simulink model "Flight_Model_2015a_07_13_2020"  (R2015a)
settings: Solver=ode45  StartTime=0.0  StopTime=120  RelTol=1e-3
model workspace (MAT data in the model file):
  rocketDiam = 0.197
  noseLength = 0.5
  totalImpulse = 10831
  finSpan = 0.4
  finArea = 0.2
  finChordAngle = 0.5236
  refArea = 0.0182
  rocketCP = 1
  bodyLength = 5
  propMass = 7.183
  gravity = 9.8067
  time = [0; 0.045; 0.067; 0.084; 0.124; 0.186; 0.231; 0.298; 0.371; 0.534; 0.979; 1.142; 2.002; 2.289; 2.761; 3.121; 3.436; 3.678; 3.79; 4.004; 4.415; 4.538; 4.656; 4.82; 5.005; 5.219; 5.371]
  thrust = [0; 2638.366; 2528.97; 3063.078; 2426.009; 2548.275; 2599.755; 2554.71; 2644.801; 2638.366; 2561.145; 2606.19; 2638.366; 2638.366; 2580.45; 2496.795; 2335.919; 2213.653; 2129.998; 1653.805; 888.035; 630.634; 450.453; 289.577; 135.136; 25.74; 0]
  wetCG = 2.1
  dryCG = 1.9
  wetMass = 30
  dryMass = 23
  brakesOn = 1
  vehicleCd = 0.8
  fullBrakesOn = 0
  brakesCd = 1
  targetAlt = 3048
undefined symbols (not defined in the file): Earth, WGS84
libraries: aerolibasang x4, aerolibbdyn x3, aerolibwind2 x2, aerolib6dof2 x2, aerospace x1, aerolibtransform2 x1, aerolibfltsims x1, aerolibatmos2 x1
settings Model: Creator=jacob  LastModifiedBy=alhus

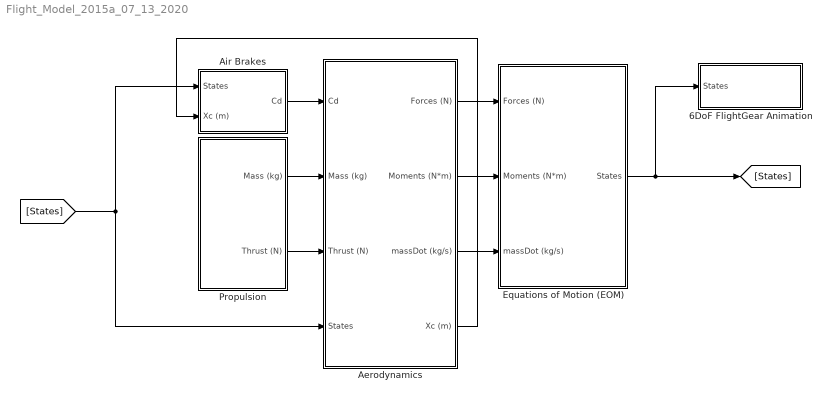
== system Flight_Model_2015a_07_13_2020 ==
  6DoF FlightGear Animation : Subsystem
  Aerodynamics : Subsystem
  Air Brakes : Subsystem
  Equations of Motion (EOM) : Subsystem
  Propulsion : Subsystem
  wires:
  Aerodynamics/1(Forces (N)) -> Equations of Motion (EOM)/1(Forces (N))
  Aerodynamics/2(Moments (N*m)) -> Equations of Motion (EOM)/2(Moments (N*m))
  Propulsion/1(Mass (kg)) -> Aerodynamics/2(Mass (kg))
  Propulsion/2(Thrust (N)) -> Aerodynamics/3(Thrust (N))
  Air Brakes/1("Cd ") -> Aerodynamics/1(Cd)
  Equations of Motion (EOM)/1(States) -> [States], 6DoF FlightGear Animation/1(States)
  [States] -> Air Brakes/1(States), Aerodynamics/4(States)
  Aerodynamics/3(massDot (kg/s)) -> Equations of Motion (EOM)/3(massDot (kg/s))
  Aerodynamics/4(Xc (m)) -> Air Brakes/2(Xc (m))

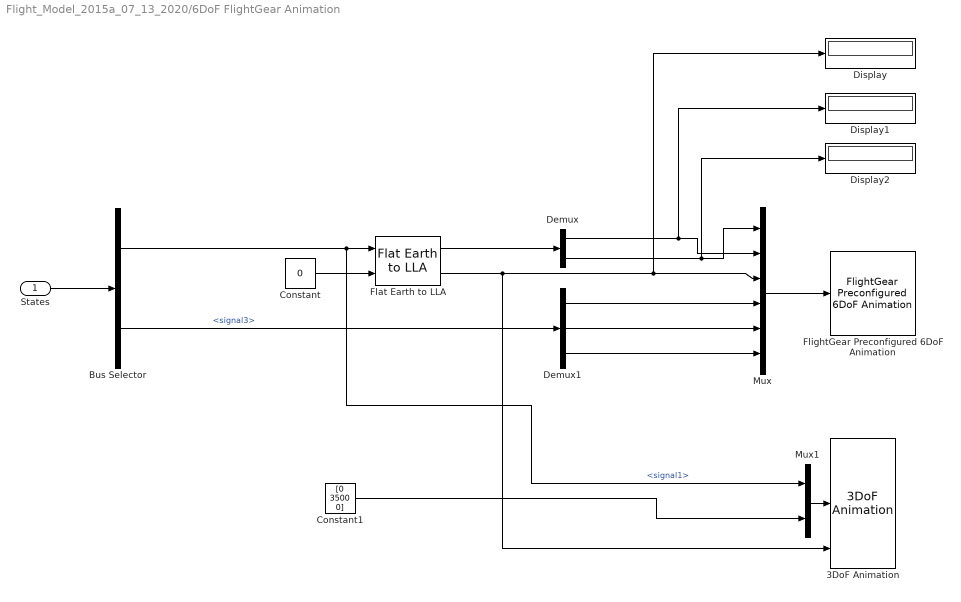
== system Flight_Model_2015a_07_13_2020/6DoF FlightGear Animation ==
  States : Inport
  3DoF Animation : aerospace/Animation/3DoF Animation  u1=[0 5000 -2000 2000 -5050 -3050]  u2=0.03  u3=1.8  u5=Fly alongside  u6=[200 200 -50]  u7=20  u8=on
  Bus Selector : BusSelector  OutputSignals=signal1,signal3
  Constant : Constant  Value=0
  Constant1 : Constant  Value=[0 3500 0]
  Demux : Demux  Outputs=2
  Demux1 : Demux  Outputs=3
  Display : Display
  Display1 : Display
  Display2 : Display
  Flat Earth to LLA : aerolibtransform2/Flat Earth to LLA  units=Metric (MKS)  ptype=Earth (WGS84)  F=1/298.257223563  R=6378137  LL0=[0 10]  psi=0
  FlightGear Preconfigured 6DoF Animation : aerolibfltsims/FlightGear Preconfigured 6DoF Animation  xFlightGearVersion=v3.0  DestinationIpAddress=127.0.0.1  DestinationPort=5502  SampleTime=1/30
  Mux : Mux  Inputs=6
  Mux1 : Mux  Inputs=2
  wires:
  States/1 -> Bus Selector/1
  Constant/1 -> Flat Earth to LLA/2
  Mux/1 -> FlightGear Preconfigured 6DoF Animation/1
  Flat Earth to LLA/1 -> Demux/1
  Demux/1 -> Display1/1, Mux/2
  Demux/2 -> Display2/1, Mux/1
  Flat Earth to LLA/2 -> 3DoF Animation/3, Display/1, Mux/3
  Demux1/2 -> Mux/5
  Demux1/3 -> Mux/6
  Demux1/1 -> Mux/4
  Bus Selector/1 -> Mux1/1, Flat Earth to LLA/1  "<signal1>"
  Bus Selector/2 -> Demux1/1  "<signal3>"
  Mux1/1 -> 3DoF Animation/2
  Constant1/1 -> Mux1/2

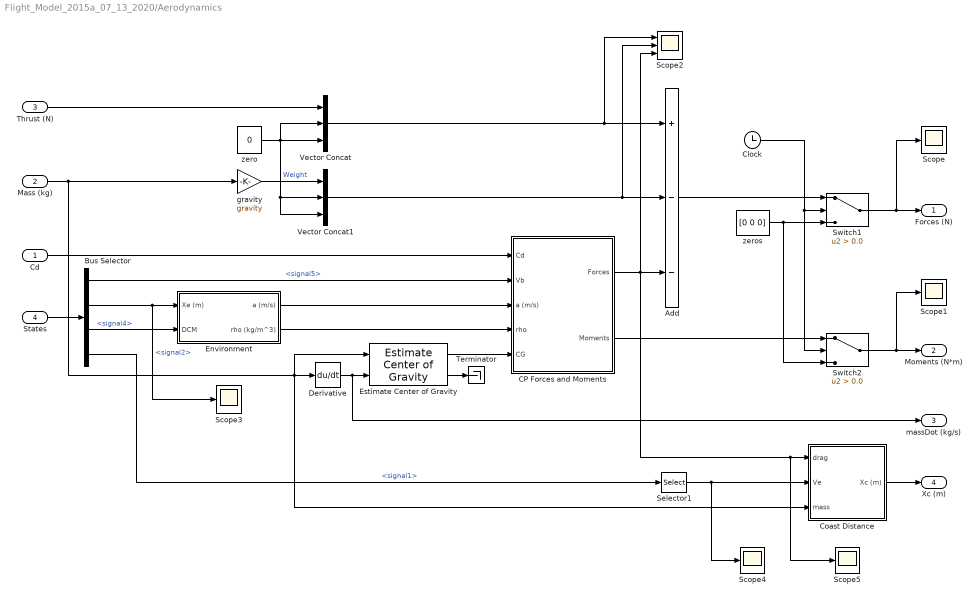
== system Flight_Model_2015a_07_13_2020/Aerodynamics ==
  Cd : Inport
  Mass (kg) : Inport  Port=2
  Thrust (N) : Inport  Port=3
  States : Inport  Port=4
  Add : Sum  Inputs=+--
  Bus Selector : BusSelector  OutputSignals=signal5,signal2,signal4,signal1
  CP Forces and Moments : Subsystem
  Clock : Clock
  Coast Distance : Subsystem
  Derivative : Derivative
  Environment : Subsystem
  Estimate Center of Gravity : aerolibbdyn/Estimate Center of Gravity  fmass=wetMass  emass=dryMass  fcg=[wetCG 0 0]'  ecg=[dryCG 0 0]'
  Scope{,1,3..5} (5 alike) : Scope
      Scope settings: YMin=-1  YMax=1  SaveName=ScopeData10
      Scope1 settings: SaveName=ScopeData11
      Scope3 settings: SaveName=ScopeData18
      Scope4 settings: SaveName=ScopeData20
      Scope5 settings: SaveName=ScopeData21
  Scope2 : Scope  NumInputPorts=3
      settings: YMin=-5~-5~-5  YMax=5~5~5  SaveName=ScopeData14
  Selector1 : Selector  InputPortWidth=3
  Switch1 : Switch  Criteria=u2 > Threshold  Threshold=0.0
  Switch2 : Switch  Criteria=u2 > Threshold  Threshold=0.0
  Terminator : Terminator
  Vector Concat : Concatenate  NumInputs=3
  Vector Concat1 : Concatenate  NumInputs=3
  gravity : Gain  Gain=gravity
  "zero " : Constant  Value=0
  "zeros " : Constant  Value=[0 0 0]
  Forces (N) : Outport
  Moments (N*m) : Outport  Port=2
  massDot (kg/s) : Outport  Port=3
  Xc (m) : Outport  Port=4
  wires:
  Mass (kg)/1 -> Coast Distance/3(mass), Estimate Center of Gravity/1, Derivative/1, gravity/1
  Derivative/1 -> Estimate Center of Gravity/2, massDot (kg/s)/1
  Estimate Center of Gravity/2 -> Terminator/1
  Estimate Center of Gravity/1 -> CP Forces and Moments/5(CG)
  Cd/1 -> CP Forces and Moments/1(Cd)
  Environment/2(rho (kg/m^3)) -> CP Forces and Moments/4(rho)
  Add/1 -> Switch1/1
  Switch1/1 -> Scope/1, Forces (N)/1
  "zeros "/1 -> Switch2/3, Switch1/3
  Clock/1 -> Switch2/2, Switch1/2
  Switch2/1 -> Scope1/1, Moments (N*m)/1
  States/1 -> Bus Selector/1
  Environment/1(a (m/s)) -> CP Forces and Moments/3(a (m/s))
  Bus Selector/1 -> CP Forces and Moments/2(Vb)  "<signal5>"
  Bus Selector/2 -> Environment/1(Xe (m)), Scope3/1  "<signal2>"
  Bus Selector/3 -> Environment/2(DCM)  "<signal4>"
  "zero "/1 -> Vector Concat/2, Vector Concat/3, Vector Concat1/2, Vector Concat1/3
  Thrust (N)/1 -> Vector Concat/1
  Vector Concat/1 -> Scope2/1, Add/1
  Vector Concat1/1 -> Scope2/2, Add/2
  CP Forces and Moments/2(Moments) -> Switch2/1
  gravity/1 -> Vector Concat1/1  "Weight"
  CP Forces and Moments/1(Forces) -> Scope5/1, Coast Distance/1(drag), Add/3, Scope2/3
  Bus Selector/4 -> Selector1/1  "<signal1>"
  Coast Distance/1(Xc (m)) -> Xc (m)/1
  Selector1/1 -> Coast Distance/2(Ve), Scope4/1

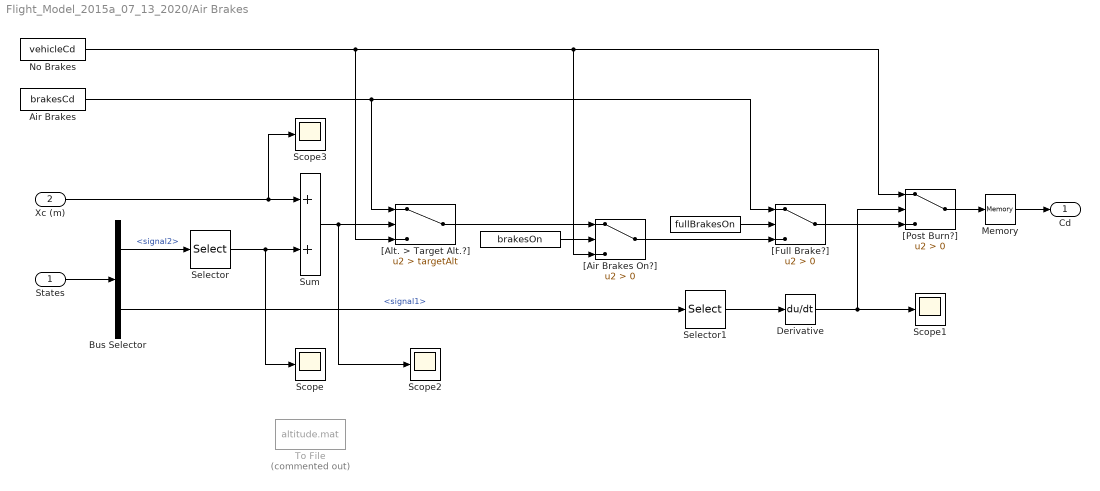
== system Flight_Model_2015a_07_13_2020/Air Brakes ==
  States : Inport
  Xc (m) : Inport  Port=2
  " " : Constant  Value=fullBrakesOn
  "  " : Constant  Value=brakesOn
  Air Brakes : Constant  Value=brakesCd
  Bus Selector : BusSelector  OutputSignals=signal2,signal1
  Derivative : Derivative
  Memory : Memory
  No Brakes : Constant  Value=vehicleCd
  Scope{,1..3} (4 alike) : Scope
      Scope settings: TimeRange=0.6678756958057797  YMin=3027.687329665507  YMax=3055.870394376453  SaveName=ScopeData4
      Scope1 settings: TimeRange=19  YMin=0  YMax=325  SaveName=ScopeData19
      Scope2 settings: TimeRange=19  YMin=0  YMax=3000  SaveName=ScopeData2
      Scope3 settings: TimeRange=19  YMin=0  YMax=2000  SaveName=ScopeData22
  "Selector " : Selector  InputPortWidth=3
  Selector1 : Selector  InputPortWidth=3
  Sum : Sum
  To File : ToFile  Commented=on  Filename=altitude.mat  SaveFormat=Timeseries
  "[Air Brakes On?]" : Switch  Description=[Air Brakes On?]  Criteria=u2 > Threshold
  "[Alt. > Target Alt.?]" : Switch  Criteria=u2 > Threshold  Threshold=targetAlt
  "[Full Brake?]" : Switch  Criteria=u2 > Threshold
  "[Post Burn?]" : Switch  Criteria=u2 > Threshold
  "Cd " : Outport
  wires:
  Sum/1 -> Scope2/1, "[Alt. > Target Alt.?]"/2
  "[Post Burn?]"/1 -> Memory/1
  No Brakes/1 -> "[Alt. > Target Alt.?]"/3, "[Post Burn?]"/1, "[Air Brakes On?]"/3
  " "/1 -> "[Full Brake?]"/2
  Air Brakes/1 -> "[Alt. > Target Alt.?]"/1, "[Full Brake?]"/1
  "[Full Brake?]"/1 -> "[Post Burn?]"/3
  "Selector "/1 -> Scope/1, Sum/2
  "  "/1 -> "[Air Brakes On?]"/2
  "[Air Brakes On?]"/1 -> "[Full Brake?]"/3
  "[Alt. > Target Alt.?]"/1 -> "[Air Brakes On?]"/1
  States/1 -> Bus Selector/1
  Selector1/1 -> Derivative/1
  Derivative/1 -> "[Post Burn?]"/2, Scope1/1
  Bus Selector/1 -> "Selector "/1  "<signal2>"
  Xc (m)/1 -> Scope3/1, Sum/1
  Bus Selector/2 -> Selector1/1  "<signal1>"
  Memory/1 -> "Cd "/1

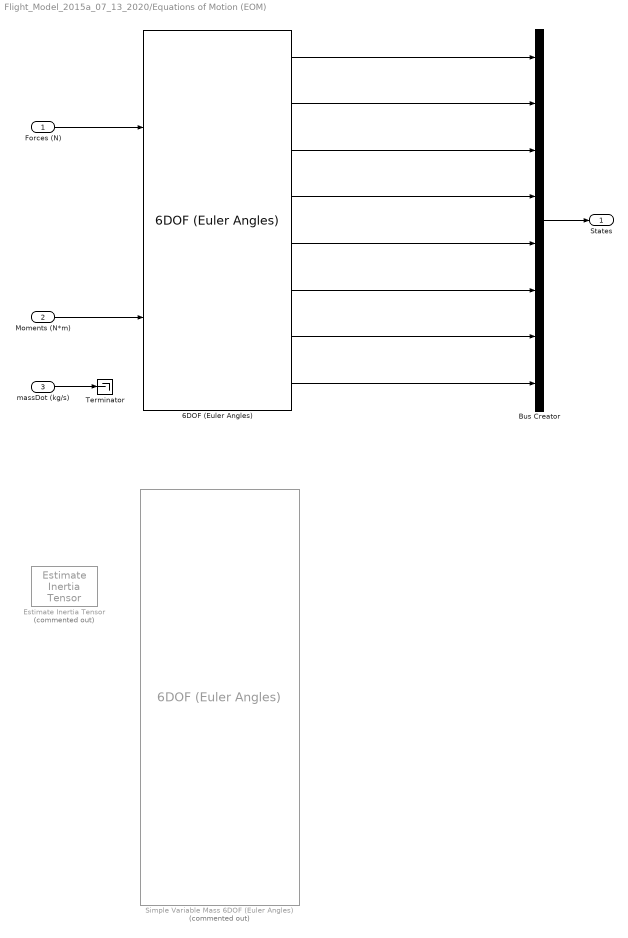
== system Flight_Model_2015a_07_13_2020/Equations of Motion (EOM) ==
  Forces (N) : Inport
  Moments (N*m) : Inport  Port=2
  massDot (kg/s) : Inport  Port=3
  6DOF (Euler Angles) : aerolib6dof2/6DOF (Euler Angles)  units=Metric (MKS)  mtype=Fixed  rep=Euler Angles  xme_0=[0 0 0]  Vm_0=[0 0 0]  eul_0=[0 0 0]  pm_0=[0, 0, 0]  mass_0=30  mass_e=0.5  mass_f=2.0  inertia=eye(3)  inertia_e=eye(3)  inertia_f=2*eye(3)  k_quat=1.0  vre_flag=on
  Bus Creator : BusCreator  Inputs=8
  Estimate Inertia Tensor : aerolibbdyn/Estimate Inertia Tensor  Commented=on  fmass=2  emass=1  fI=eye(3)  eI=eye(3)/2
  Simple Variable Mass 6DOF (Euler Angles) : aerolib6dof2/6DOF (Euler Angles)  Commented=on  units=Metric (MKS)  mtype=Simple Variable  rep=Euler Angles  xme_0=[0 0 0]  Vm_0=[0 0 0]  eul_0=[0 0 0]  pm_0=[0 0 0]  mass_0=1.0  mass_e=0.5  mass_f=2.0  inertia=eye(3)  inertia_e=eye(3)  inertia_f=2*eye(3)  k_quat=1.0  vre_flag=off
  Terminator : Terminator
  States : Outport
  wires:
  Forces (N)/1 -> 6DOF (Euler Angles)/1
  6DOF (Euler Angles)/2 -> Bus Creator/2
  6DOF (Euler Angles)/1 -> Bus Creator/1
  Bus Creator/1 -> States/1
  6DOF (Euler Angles)/3 -> Bus Creator/3
  6DOF (Euler Angles)/4 -> Bus Creator/4
  6DOF (Euler Angles)/5 -> Bus Creator/5
  6DOF (Euler Angles)/6 -> Bus Creator/6
  6DOF (Euler Angles)/7 -> Bus Creator/7
  6DOF (Euler Angles)/8 -> Bus Creator/8
  massDot (kg/s)/1 -> Terminator/1
  Moments (N*m)/1 -> 6DOF (Euler Angles)/2

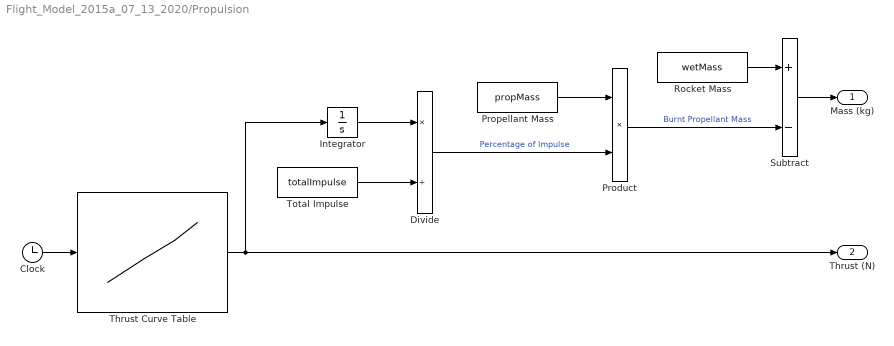
== system Flight_Model_2015a_07_13_2020/Propulsion ==
  Clock : Clock
  Divide : Product  Inputs=*/
  Integrator : Integrator
  Product : Product
  Propellant Mass : Constant  Value=propMass
  Rocket Mass : Constant  Value=wetMass
  Subtract : Sum  Inputs=+-
  Thrust Curve Table : Lookup_n-D  NumberOfTableDimensions=1  BreakpointsForDimension1=time  Table=thrust  ExtrapMethod=Clip  InternalRulePriority=Speed  RndMeth=Simplest  InputSameDT=on
  Total Impulse : Constant  Value=totalImpulse
  Mass (kg) : Outport
  Thrust (N) : Outport  Port=2
  wires:
  Total Impulse/1 -> Divide/2
  Integrator/1 -> Divide/1
  Clock/1 -> Thrust Curve Table/1
  Propellant Mass/1 -> Product/1
  Product/1 -> Subtract/2  "Burnt Propellant Mass"
  Rocket Mass/1 -> Subtract/1
  Subtract/1 -> Mass (kg)/1
  Thrust Curve Table/1 -> Thrust (N)/1, Integrator/1
  Divide/1 -> Product/2  "Percentage of Impulse"

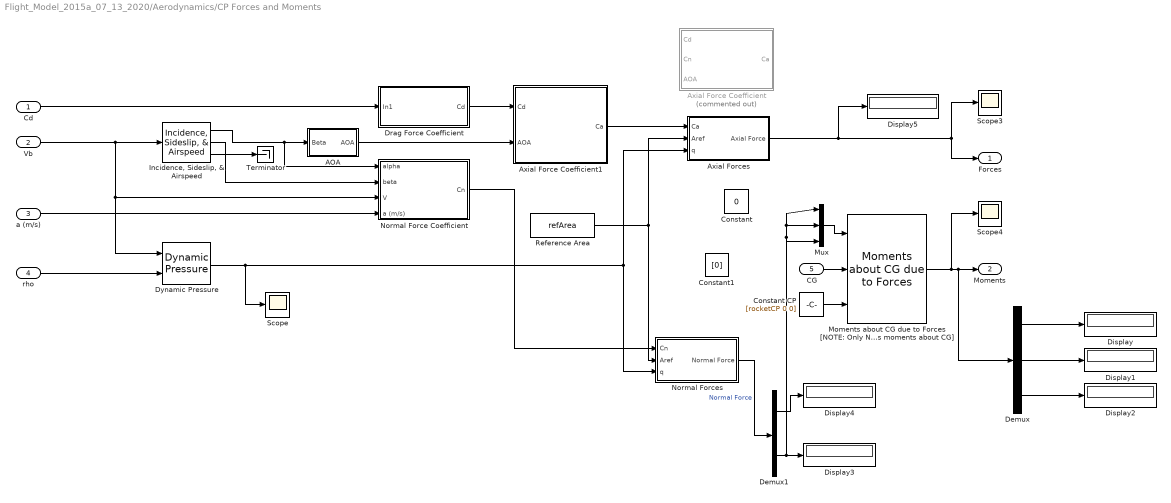
== system Flight_Model_2015a_07_13_2020/Aerodynamics/CP Forces and Moments ==
  Cd : Inport
  Vb : Inport  Port=2
  a (m/s) : Inport  Port=3
  rho : Inport  Port=4
  CG : Inport  Port=5
  AOA : Subsystem
  Axial Force Coefficient : Subsystem  Commented=on
  Axial Force Coefficient1 : Subsystem
  Axial Forces : Subsystem
  Constant : Constant  Value=0
  Constant CP : Constant  Value=[rocketCP 0 0]
  Constant1 : Constant  Value=[0]
  Demux : Demux  Outputs=3
  Demux1 : Demux  Outputs=2
  Display{,1..5} (6 alike) : Display
  Drag Force Coefficient : Subsystem
  Dynamic Pressure : aerolibasang/Dynamic Pressure
  "Incidence, Sideslip, & Airspeed" : aerolibasang/Incidence, Sideslip, & Airspeed
  Moments about CG due to Forces [NOTE: Only Normal Force applys moments about CG] : aerolibbdyn/Moments about CG  due to Forces
  Mux : Mux  Inputs=3
  Normal Force Coefficient : Subsystem
  Normal Forces : Subsystem
  Reference Area : Constant  Value=refArea
  Scope : Scope
      settings: SaveName=ScopeData9
  Scope3 : Scope
      settings: SaveName=ScopeData7
  Scope4 : Scope
      settings: SaveName=ScopeData8
  Terminator : Terminator
  Forces : Outport
  Moments : Outport  Port=2
  wires:
  CG/1 -> Moments about CG due to Forces [NOTE: Only Normal Force applys moments about CG]/2
  Vb/1 -> Dynamic Pressure/1, Normal Force Coefficient/3(V), "Incidence, Sideslip, & Airspeed"/1
  Drag Force Coefficient/1(Cd) -> Axial Force Coefficient1/1(Cd)
  Axial Force Coefficient1/1(Ca) -> Axial Forces/1(Ca)
  Axial Forces/1(Axial Force) -> Display5/1, Forces/1, Scope3/1
  rho/1 -> Dynamic Pressure/2
  a (m/s)/1 -> Normal Force Coefficient/4(a (m/s))
  Dynamic Pressure/1 -> Scope/1, Normal Forces/3("q "), Axial Forces/3("q ")
  AOA/1(AOA) -> Axial Force Coefficient1/2(AOA)
  Cd/1 -> Drag Force Coefficient/1(In1)
  Reference Area/1 -> Normal Forces/2(Aref), Axial Forces/2(Aref)
  Constant CP/1 -> Moments about CG due to Forces [NOTE: Only Normal Force applys moments about CG]/3
  Moments about CG due to Forces [NOTE: Only Normal Force applys moments about CG]/1 -> Scope4/1, Demux/1, Moments/1
  "Incidence, Sideslip, & Airspeed"/1 -> Normal Force Coefficient/1(alpha), AOA/1(Beta)
  "Incidence, Sideslip, & Airspeed"/2 -> Normal Force Coefficient/2(beta)
  "Incidence, Sideslip, & Airspeed"/3 -> Terminator/1
  Demux/1 -> Display/1
  Demux/2 -> Display1/1
  Demux/3 -> Display2/1
  Mux/1 -> Moments about CG due to Forces [NOTE: Only Normal Force applys moments about CG]/1
  Normal Force Coefficient/1(Cn) -> Normal Forces/1(Cn)
  Demux1/2 -> Mux/1, Mux/2, Mux/3, Display3/1
  Normal Forces/1(Normal Force) -> Demux1/1  "Normal Force"
  Demux1/1 -> Display4/1

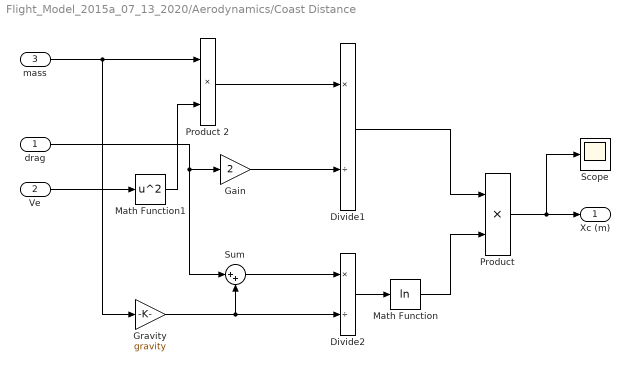
== system Flight_Model_2015a_07_13_2020/Aerodynamics/Coast Distance ==
  drag : Inport
  Ve : Inport  Port=2
  mass : Inport  Port=3
  Divide1 : Product  Inputs=*/
  Divide2 : Product  Inputs=*/
  Gain : Gain  Gain=2
  Gravity : Gain  Gain=gravity
  Math Function : Math  Operator=log  SaturateOnIntegerOverflow=on
  Math Function1 : Math  Operator=square  SaturateOnIntegerOverflow=on
  Product : Product
  Product 2 : Product  Inputs=**
  Scope : Scope
      settings: SaveName=ScopeData50
  Sum : Sum  Inputs=|++
  Xc (m) : Outport
  wires:
  Math Function/1 -> Product/2
  mass/1 -> Gravity/1, Product 2/1
  Divide1/1 -> Product/1
  drag/1 -> Gain/1, Sum/1
  Divide2/1 -> Math Function/1
  Product/1 -> Xc (m)/1, Scope/1
  Sum/1 -> Divide2/1
  Gravity/1 -> Sum/2, Divide2/2
  Ve/1 -> Math Function1/1
  Math Function1/1 -> Product 2/2
  Product 2/1 -> Divide1/1
  Gain/1 -> Divide1/2

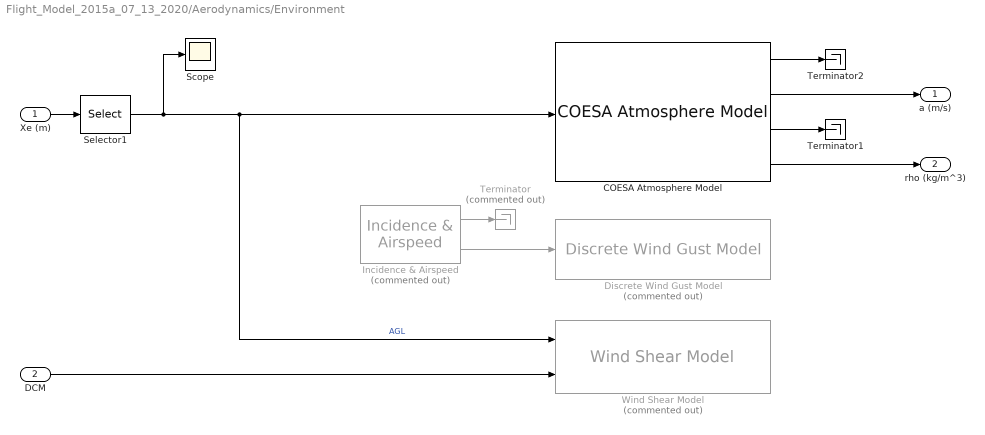
== system Flight_Model_2015a_07_13_2020/Aerodynamics/Environment ==
  Xe (m) : Inport
  DCM : Inport  Port=2
  COESA Atmosphere Model : aerolibatmos2/COESA Atmosphere Model  units=Metric (MKS)  spec=1976 COESA-extended U.S. Standard Atmosphere  model=Profile  profile_var=High temperature  profile_percent=1%  profile_alt=5 km (16404 ft)  envelope_var=High temperature  envelope_percent=1%  action=Warning
  Discrete Wind Gust Model : aerolibwind2/Discrete Wind Gust Model  Commented=on  units=Metric (MKS)  Gx=on  Gy=on  Gz=on  t_0=5  d_m=[120 120 80]  v_m=[3.5 3.5 3.0]
  Incidence & Airspeed : aerolibasang/Incidence  & Airspeed  Commented=on
  Scope : Scope
      settings: SaveName=ScopeData12
  Selector1 : Selector  InputPortWidth=3  Indices=3
  Terminator : Terminator  Commented=on
  Terminator1 : Terminator
  Terminator2 : Terminator
  Wind Shear Model : aerolibwind2/Wind Shear Model  Commented=on  units=Metric (MKS)  phase=Category C - Terminal Flight Phase  W_20=15  Wdeg=0
  a (m/s) : Outport
  rho (kg/m^3) : Outport  Port=2
  wires:
  Incidence & Airspeed/2 -> Discrete Wind Gust Model/1
  Incidence & Airspeed/1 -> Terminator/1
  Xe (m)/1 -> Selector1/1
  DCM/1 -> Wind Shear Model/2
  Selector1/1 -> Wind Shear Model/1, COESA Atmosphere Model/1, Scope/1  "AGL"
  COESA Atmosphere Model/2 -> a (m/s)/1
  COESA Atmosphere Model/4 -> rho (kg/m^3)/1
  COESA Atmosphere Model/1 -> Terminator2/1
  COESA Atmosphere Model/3 -> Terminator1/1

== system Flight_Model_2015a_07_13_2020/Aerodynamics/CP Forces and Moments/AOA ==
  Beta : Inport
  AOA : Outport
  wires:
  Beta/1 -> AOA/1

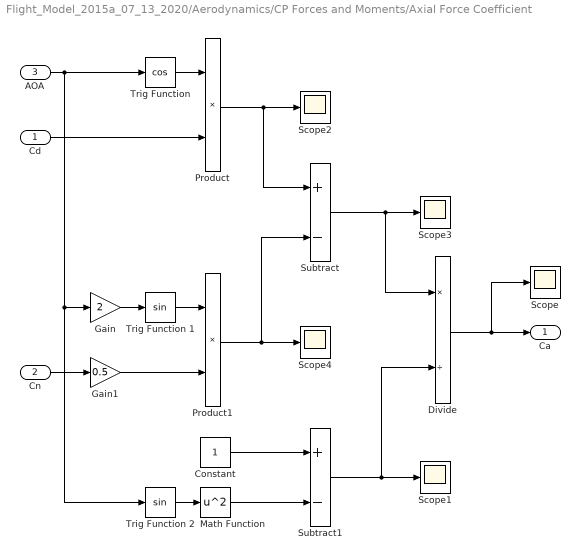
== system Flight_Model_2015a_07_13_2020/Aerodynamics/CP Forces and Moments/Axial Force Coefficient ==
  Cd : Inport
  Cn : Inport  Port=2
  AOA : Inport  Port=3
  Constant : Constant
  Divide : Product  Inputs=*/
  Gain : Gain  Gain=2
  Gain1 : Gain  Gain=0.5
  Math Function : Math  Operator=square  SaturateOnIntegerOverflow=on
  Product : Product
  Product1 : Product
  Scope{,1..4} (5 alike) : Scope
      Scope settings: SaveName=ScopeData5
      Scope1 settings: SaveName=ScopeData13
      Scope2 settings: SaveName=ScopeData15
      Scope3 settings: SaveName=ScopeData16
      Scope4 settings: SaveName=ScopeData17
  Subtract : Sum  Inputs=+-
  Subtract1 : Sum  Inputs=+-
  Trig Function : Trigonometry  Operator=cos
  Trig Function 1 : Trigonometry
  Trig Function 2 : Trigonometry
  Ca : Outport
  wires:
  AOA/1 -> Trig Function/1, Trig Function 2/1, Gain/1
  Cd/1 -> Product/2
  Trig Function/1 -> Product/1
  Gain/1 -> Trig Function 1/1
  Trig Function 1/1 -> Product1/1
  Gain1/1 -> Product1/2
  Cn/1 -> Gain1/1
  Product1/1 -> Scope4/1, Subtract/2
  Divide/1 -> Scope/1, Ca/1
  Trig Function 2/1 -> Math Function/1
  Math Function/1 -> Subtract1/2
  Constant/1 -> Subtract1/1
  Subtract/1 -> Scope3/1, Divide/1
  Subtract1/1 -> Scope1/1, Divide/2
  Product/1 -> Scope2/1, Subtract/1

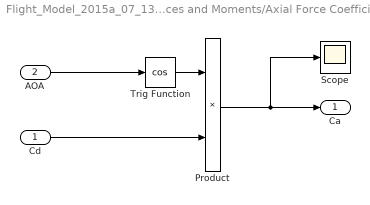
== system Flight_Model_2015a_07_13_2020/Aerodynamics/CP Forces and Moments/Axial Force Coefficient1 ==
  Cd : Inport
  AOA : Inport  Port=2
  Product : Product
  Scope : Scope
      settings: SaveName=ScopeData15
  Trig Function : Trigonometry  Operator=cos
  Ca : Outport
  wires:
  AOA/1 -> Trig Function/1
  Cd/1 -> Product/2
  Trig Function/1 -> Product/1
  Product/1 -> Ca/1, Scope/1

== system Flight_Model_2015a_07_13_2020/Aerodynamics/CP Forces and Moments/Axial Forces ==
  Ca : Inport
  Aref : Inport  Port=2
  "q " : Inport  Port=3
  Product : Product  Inputs=3
  Scope : Scope
      settings: TimeRange=10  YMin=-100000000  YMax=0  SaveName=ScopeData6
  Axial Force : Outport
  wires:
  Ca/1 -> Product/1
  Aref/1 -> Product/2
  Product/1 -> Axial Force/1, Scope/1
  "q "/1 -> Product/3

== system Flight_Model_2015a_07_13_2020/Aerodynamics/CP Forces and Moments/Drag Force Coefficient ==
  In1 : Inport
  Cd : Outport
  wires:
  In1/1 -> Cd/1

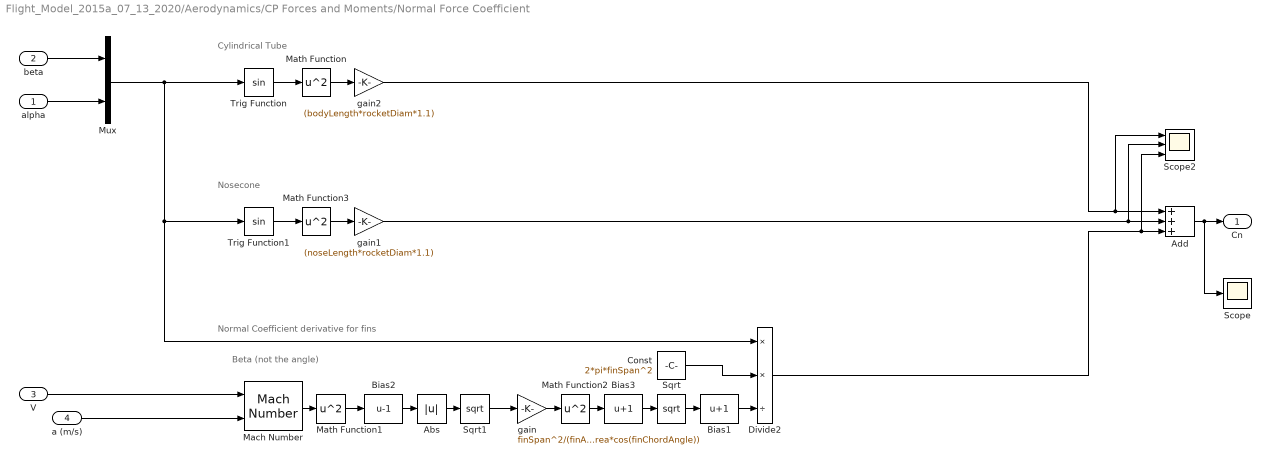
== system Flight_Model_2015a_07_13_2020/Aerodynamics/CP Forces and Moments/Normal Force Coefficient ==
  note: Cylindrical Tube
  note: Normal Coefficient derivative for fins
  note: Beta (not the angle)
  note: Nosecone
  alpha : Inport
  beta : Inport  Port=2
  V : Inport  Port=3
  a (m/s) : Inport  Port=4
  Abs : Abs
  Add : Sum  Inputs=+++
  Bias1 : Bias  Bias=1
  Bias2 : Bias  Bias=-1
  Bias3 : Bias  Bias=1
  Const : Constant  Value=2*pi*finSpan^2
  Divide2 : Product  Inputs=**/
  Mach Number : aerolibasang/Mach Number
  Math Function{,1..3} (4 alike) : Math  Operator=square  SaturateOnIntegerOverflow=on
  Mux : Mux  Inputs=2
  Scope : Scope
  Scope2 : Scope  NumInputPorts=3
      settings: YMin=-5~-5~-5  YMax=5~5~5  SaveName=ScopeData3
  Sqrt : Sqrt  SaturateOnIntegerOverflow=on
  Sqrt1 : Sqrt  SaturateOnIntegerOverflow=on
  Trig Function : Trigonometry
  Trig Function1 : Trigonometry
  gain : Gain  Gain=finSpan^2/(finArea*cos(finChordAngle))
  gain1 : Gain  Gain=(noseLength*rocketDiam*1.1)
  gain2 : Gain  Gain=(bodyLength*rocketDiam*1.1)
  Cn : Outport
  wires:
  Trig Function/1 -> Math Function/1
  Sqrt1/1 -> gain/1
  Math Function2/1 -> Bias3/1
  Sqrt/1 -> Bias1/1
  Bias3/1 -> Sqrt/1
  gain/1 -> Math Function2/1
  a (m/s)/1 -> Mach Number/2
  Bias1/1 -> Divide2/3
  Math Function/1 -> gain2/1
  Trig Function1/1 -> Math Function3/1
  Math Function3/1 -> gain1/1
  Add/1 -> Scope/1, Cn/1
  V/1 -> Mach Number/1
  Mach Number/1 -> Math Function1/1
  Math Function1/1 -> Bias2/1
  Bias2/1 -> Abs/1
  Abs/1 -> Sqrt1/1
  Mux/1 -> Divide2/1, Trig Function1/1, Trig Function/1
  Const/1 -> Divide2/2
  gain1/1 -> Scope2/2, Add/2
  gain2/1 -> Add/1, Scope2/1
  Divide2/1 -> Add/3, Scope2/3
  alpha/1 -> Mux/2
  beta/1 -> Mux/1

== system Flight_Model_2015a_07_13_2020/Aerodynamics/CP Forces and Moments/Normal Forces ==
  Cn : Inport
  Aref : Inport  Port=2
  "q " : Inport  Port=3
  Product : Product  Inputs=3
  Scope : Scope
      settings: TimeRange=10  YMin=-100000000  YMax=0  SaveName=ScopeData6
  Normal Force : Outport
  wires:
  Cn/1 -> Product/1
  Aref/1 -> Product/2
  Product/1 -> Normal Force/1, Scope/1
  "q "/1 -> Product/3
